simulink library "headingSetpointCalculation"  (R2018a)
settings: Solver=VariableStepAuto  StartTime=0.0  StopTime=10.0  RelTol=1e-3
libraries: controllerComponents x3, simulink x1
settings Model: Creator=mitch  LastModifiedBy=mitch

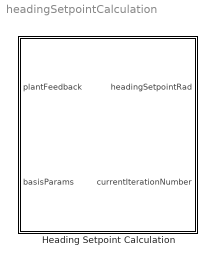
== system headingSetpointCalculation ==
  Heading Setpoint Calculation : Subsystem  VariantControl=variantPureCarrotFollowing

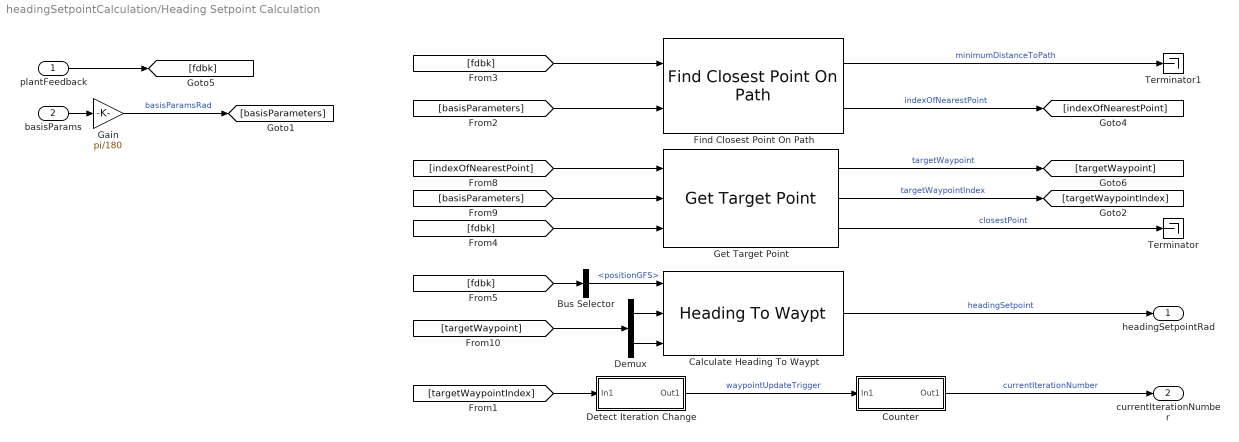
== system headingSetpointCalculation/Heading Setpoint Calculation ==
  plantFeedback : Inport  OutDataTypeStr=Bus: busPlantFeedback
  basisParams : Inport  Port=2
  Bus Selector : BusSelector  OutputSignals=positionGFS
  Calculate Heading To Waypt : controllerComponents/Heading To Waypt
  Counter : Subsystem
  Demux : Demux  Outputs=2
  Detect Iteration Change : Subsystem
  Find Closest Point On Path : controllerComponents/Find Closest Point On Path
  Gain : Gain  Gain=pi/180
  Get Target Point : controllerComponents/Get Target Point
  Terminator : Terminator
  Terminator1 : Terminator
  headingSetpointRad : Outport
  currentIterationNumber : Outport  Port=2
  wires:
  Get Target Point/3 -> Terminator/1  "closestPoint"
  plantFeedback/1 -> [fdbk]
  Get Target Point/2 -> [targetWaypointIndex]  "targetWaypointIndex"
  Detect Iteration Change/1(Out1) -> Counter/1(In1)  "waypointUpdateTrigger"
  Counter/1(Out1) -> currentIterationNumber/1  "currentIterationNumber"
  [targetWaypointIndex] -> Detect Iteration Change/1(In1)
  Calculate Heading To Waypt/1 -> headingSetpointRad/1  "headingSetpoint"
  [targetWaypoint] -> Demux/1
  Get Target Point/1 -> [targetWaypoint]  "targetWaypoint"
  [basisParameters] -> Get Target Point/2
  [indexOfNearestPoint] -> Get Target Point/1
  Find Closest Point On Path/2 -> [indexOfNearestPoint]  "indexOfNearestPoint"
  Find Closest Point On Path/1 -> Terminator1/1  "minimumDistanceToPath"
  Demux/2 -> Calculate Heading To Waypt/3
  Demux/1 -> Calculate Heading To Waypt/2
  [basisParameters] -> Find Closest Point On Path/2
  [fdbk] -> Find Closest Point On Path/1
  [fdbk] -> Get Target Point/3
  basisParams/1 -> Gain/1
  [fdbk] -> Bus Selector/1
  Bus Selector/1 -> Calculate Heading To Waypt/1  "<positionGFS>"
  Gain/1 -> [basisParameters]  "basisParamsRad"

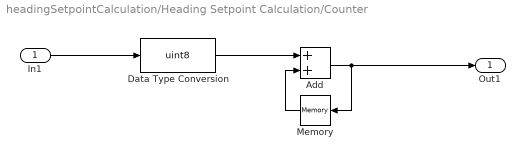
== system headingSetpointCalculation/Heading Setpoint Calculation/Counter ==
  In1 : Inport
  Add : Sum
  Data Type Conversion : DataTypeConversion  OutDataTypeStr=uint8
  Memory : Memory  InitialCondition=1
  Out1 : Outport  OutDataTypeStr=double
  wires:
  Data Type Conversion/1 -> Add/1
  In1/1 -> Data Type Conversion/1
  Memory/1 -> Add/2
  Add/1 -> Memory/1, Out1/1

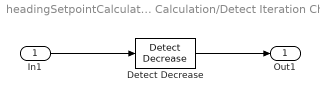
== system headingSetpointCalculation/Heading Setpoint Calculation/Detect Iteration Change ==
  In1 : Inport
  Detect Decrease : simulink/Logic and Bit Operations/Detect Decrease  vinit=0.0  OutDataTypeStr=boolean
  Out1 : Outport
  wires:
  Detect Decrease/1 -> Out1/1
  In1/1 -> Detect Decrease/1
